simulink model "powerlib_utilityV2"  (Simulink 6.0)
settings: Solver=VariableStepDiscrete  SolverMode=SingleTasking  StartTime=0.0  StopTime=10.0  RelTol=1e-3  AbsTol=1e-6
settings Model: Creator=patrice  LastModifiedBy=batserve  ExtModeTrigMode=oneshot  ExtModeArmWhenConnect=off  ExtModeAutoUpdateStatusClock=off
settings DataIOCC: LimitDataPoints=off  SignalLoggingName=sigsOut
settings OptimizationCC: BlockReduction=off  BooleanDataType=off
settings DebuggingCC: SolverPrmCheckMsg=none  UnconnectedInputMsg=none  UnconnectedOutputMsg=none
settings HardwareCC: TargetUnknown=on
settings RTWCC: TemplateMakefile=grt_unix.tmf

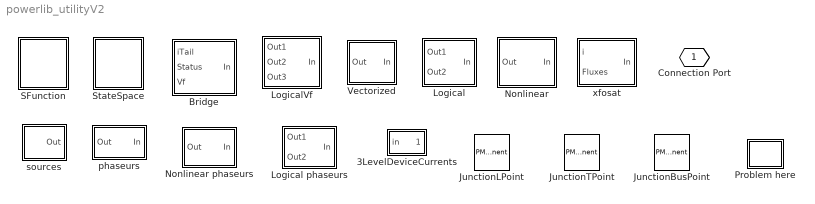
== system powerlib_utilityV2 ==
  3LevelDeviceCurrents : Subsystem  mask(Determine device currents){nb_arm=3}
      mask prompts: nb_arm "Number of arms:"
      mask init:
      | if nb_arm==1,
      |    ImesElements1=[1:3];
      |    ImesElements2=[1:10];
      | elseif nb_arm==2,
      |    ImesElements1=[1 4 2 5 3 6];
      |    ImesElements2=[1:2:19 2:2:20];
      | elseif nb_arm==3,
      |    ImesElements1=[1 4 7 2 5 8 3 6 9];
      |    ImesElements2=[1:3:28 2:3:29 3:3:30];
      | end
  Bridge : Subsystem  Orientation=left
  JunctionBusPoint : PMComponent  Tag=PoWeRsYsTeMbLoCk  PhysicalDomain=powersysdomain  LeftPortType=p1  RightPortType=p1  LConnTagsString=I1|I2  RConnTagsString=O1|O2  mask(JunctionPoint){entrees=2, sorties=2}
      mask prompts: entrees "inputs"; sorties "outputs"
      mask help: This block is used to replace the Bus Bar block from powerlib2. This block was generated by the psbupdate function. With SimPowerSystems, this block is not required. You should consider deleting this block and reconnect the lines together.
      mask init:
      | inputtags = cell(1,entrees);
      | 
      | for i=1:entrees
      | 
      | 	inputtags{i} = ['I',num2str(i)];
      | 
      | end
      | 
      | outputtags = cell(1,sorties);
      | 
      | for i=1:sorties
      | 
      | 	outputtags{i} = ['O',num2str(i)];
      | 
      | end
      | 
      | set_param(gcbh,'LConnTags',inputtags);
      | 
      | set_param(gcbh,'RConnTags',outputtags);
      mask Display:
      | color('red');
      | 
      | plot([0,100],[0,100])
      | 
      | plot([0,100],[100,0])
  JunctionLPoint : PMComponent  Tag=PoWeRsYsTeMbLoCk  PhysicalDomain=powersysdomain  LeftPortType=p1  RightPortType=p1  LConnTagsString=1  RConnTagsString=__newr0
      mask Type: JunctionPoint
      mask Description: This block is used  to replace the L connector block from powerlib2. This block was generated by the psbupdate function. With SimPowerSystems, this block is not required. You should consider deleting this block and reconnect the lines together.
      mask Display:
      | color('red');
      | 
      | plot([0,100],[0,100])
      | 
      | plot([0,100],[100,0])
  JunctionTPoint : PMComponent  Tag=PoWeRsYsTeMbLoCk  PhysicalDomain=powersysdomain  LeftPortType=p1  RightPortType=p1  LConnTagsString=1|2  RConnTagsString=__newr0
      mask Type: JunctionPoint
      mask Description: This block is used  to replace the T connector block from powerlib2. This block was generated by the psbupdate function. With SimPowerSystems, this block is not required. You should consider deleting this block and reconnect the lines together.
      mask Display:
      | color('red');
      | 
      | plot([0,100],[0,100])
      | 
      | plot([0,100],[100,0])
  Logical : Subsystem  Orientation=left
  Logical phaseurs : Subsystem  Orientation=left
  LogicalVf : Subsystem  Orientation=left
  Nonlinear : Subsystem  Orientation=left
  Nonlinear phaseurs : Subsystem  Orientation=left
  Problem here : Subsystem
      mask Display: plot([-1,1,1,-1,-1],[1,1,-1,-1,1])
  SFunction : Subsystem
  StateSpace : Subsystem
  Vectorized : Subsystem  Orientation=left
  phaseurs : Subsystem  Orientation=left
  sources : Subsystem
  xfosat : Subsystem  Orientation=left
  Connection Port : PMIOPort  Tag=PMCPort  Port=1  Side=Left

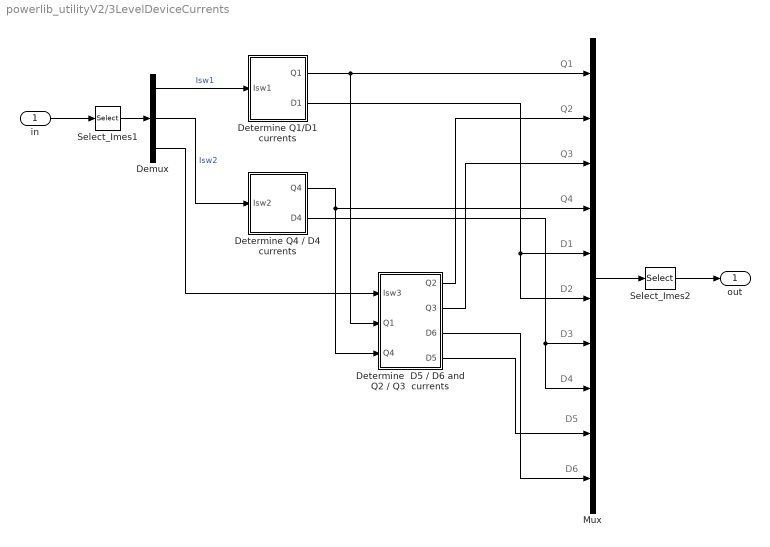
== system powerlib_utilityV2/3LevelDeviceCurrents ==
  note: Q1
  note: Q2
  note: Q3
  note: Q4
  note: D1
  note: D2
  note: D3
  note: D4
  note: D5
  note: D6
  in : Inport  Port=1  LatchInput=off
  Demux : Demux  Outputs=[nb_arm nb_arm nb_arm]
  Determine  D5 / D6 and Q2 / Q3  currents : Subsystem
  Determine Q1/D1 currents : Subsystem
  Determine Q4 / D4 currents : Subsystem
  Mux : Mux  Inputs=nb_arm*ones(10,1)
  Select_Imes1 : Selector  Elements=ImesElements1  InputPortWidth=nb_arm*3
  Select_Imes2 : Selector  Elements=ImesElements2  InputPortWidth=nb_arm*10
  out : Outport
  wires:
  Select_Imes1/1 -> Demux/1
  in/1 -> Select_Imes1/1
  Mux/1 -> Select_Imes2/1
  Select_Imes2/1 -> out/1
  Demux/1 -> Determine Q1/D1 currents/1(Isw1)  "Isw1"
  Demux/2 -> Determine Q4 / D4 currents/1(Isw2)  "Isw2"
  Demux/3 -> Determine  D5 / D6 and Q2 / Q3  currents/1(Isw3)
  Determine Q4 / D4 currents/1(Q4) -> Determine  D5 / D6 and Q2 / Q3  currents/3(Q4), Mux/4
  Determine Q1/D1 currents/1(Q1) -> Determine  D5 / D6 and Q2 / Q3  currents/2(Q1), Mux/1
  Determine  D5 / D6 and Q2 / Q3  currents/1(Q2) -> Mux/2
  Determine  D5 / D6 and Q2 / Q3  currents/2(Q3) -> Mux/3
  Determine Q1/D1 currents/2(D1) -> Mux/5, Mux/6
  Determine  D5 / D6 and Q2 / Q3  currents/3(D6) -> Mux/10
  Determine  D5 / D6 and Q2 / Q3  currents/4(D5) -> Mux/9
  Determine Q4 / D4 currents/2(D4) -> Mux/8, Mux/7

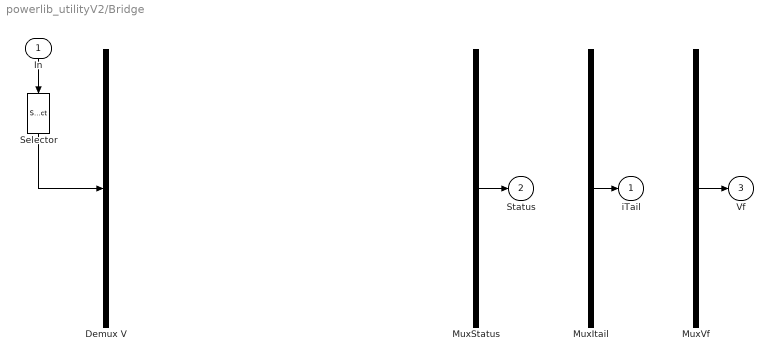
== system powerlib_utilityV2/Bridge ==
  In : Inport  Orientation=down  Port=1  LatchInput=off
  Demux V : Demux  Outputs=1
  MuxItail : Mux  Inputs=1
  MuxStatus : Mux  Inputs=1
  MuxVf : Mux  Inputs=1
  Selector : Selector  Orientation=down  InputPortWidth=1
  iTail : Outport  InitialOutput=0
  Status : Outport  Port=2  InitialOutput=0
  Vf : Outport  Port=3  InitialOutput=0
  wires:
  MuxStatus/1 -> Status/1
  MuxItail/1 -> iTail/1
  MuxVf/1 -> Vf/1
  In/1 -> Selector/1
  Selector/1 -> Demux V/1

== system powerlib_utilityV2/Logical ==
  In : Inport  Port=1  LatchInput=off
  Selector : Selector  InputPortWidth=1
  froms : Subsystem
  gotos : Subsystem
  Out1 : Outport  InitialOutput=0
  Out2 : Outport  Port=2  InitialOutput=0
  wires:
  In/1 -> Selector/1

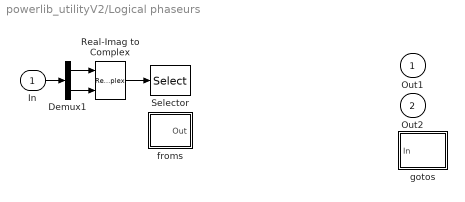
== system powerlib_utilityV2/Logical phaseurs ==
  In : Inport  Port=1  LatchInput=off
  Demux1 : Demux  Outputs=2
  Real-Imag to Complex : RealImagToComplex
  Selector : Selector  InputPortWidth=1
  froms : Subsystem
  gotos : Subsystem
  Out1 : Outport  InitialOutput=0
  Out2 : Outport  Port=2  InitialOutput=0
  wires:
  Demux1/1 -> Real-Imag to Complex/1
  Demux1/2 -> Real-Imag to Complex/2
  Real-Imag to Complex/1 -> Selector/1
  In/1 -> Demux1/1

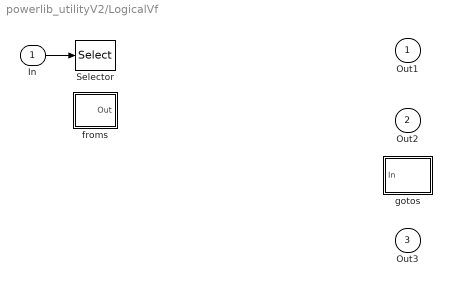
== system powerlib_utilityV2/LogicalVf ==
  In : Inport  Port=1  LatchInput=off
  Selector : Selector  InputPortWidth=1
  froms : Subsystem
  gotos : Subsystem
  Out1 : Outport  InitialOutput=0
  Out2 : Outport  Port=2  InitialOutput=0
  Out3 : Outport  Port=3  InitialOutput=0
  wires:
  In/1 -> Selector/1

== system powerlib_utilityV2/Nonlinear ==
  In : Inport  Port=1  LatchInput=off
  Demux : Demux  Outputs=1
  Mux : Mux  Inputs=1
  Selector : Selector  InputPortWidth=1
  Out : Outport  InitialOutput=0
  wires:
  In/1 -> Selector/1
  Selector/1 -> Demux/1
  Mux/1 -> Out/1

== system powerlib_utilityV2/Nonlinear phaseurs ==
  In : Inport  Port=1  LatchInput=off
  Demux : Demux  Outputs=1
  Demux1 : Demux  Outputs=2
  Mux : Mux  Inputs=1
  Real-Imag to Complex : RealImagToComplex
  Selector : Selector  InputPortWidth=1
  Out : Outport  InitialOutput=0
  wires:
  Mux/1 -> Out/1
  Selector/1 -> Demux/1
  Demux1/1 -> Real-Imag to Complex/1
  Demux1/2 -> Real-Imag to Complex/2
  In/1 -> Demux1/1
  Real-Imag to Complex/1 -> Selector/1

== system powerlib_utilityV2/Problem here ==
  note: This block identifies a connection problem
      | during the update of the model

== system powerlib_utilityV2/SFunction ==
  phaseurs : Subsystem
      mask init:
      | H=0;Rswitch=1;
  phaseursNoVf : Subsystem
      mask init:
      | H=0;Rswitch=1;
  structure : Subsystem
      mask init:
      | A=0;B=0;C=0;D=0;x0=0;Rswitch=1;TypeSwitch=0;Ts=0;YSwitchCurrent=-1;
  structureNoVf : Subsystem
      mask init:
      | A=0;B=0;C=0;D=0;x0=0;Rswitch=1;TypeSwitch=0;Ts=0;YSwitchCurrent=-1;

== system powerlib_utilityV2/StateSpace ==
  phaseurs : Subsystem
      mask init:
      | H=0;Rswitch=1;
  phaseursNoVf : Subsystem
      mask init:
      | H=0;Rswitch=1;
  structure1 : Subsystem
      mask init:
      | A=0;B=0;C=0;D=0;x0=0;Rswitch=1;TypeSwitch=0;Ts=0;
  structure1Discrete : Subsystem
      mask init:
      | A=0;B=0;C=0;D=0;x0=0;Rswitch=1;TypeSwitch=0;Ts=0;
  structure2 : Subsystem
      mask init:
      | A=0;B=0;C=0;D=0;x0=0;Rswitch=1;TypeSwitch=0;Ts=0;
  structure2Discrete : Subsystem
      mask init:
      | A=0;B=0;C=0;D=0;x0=0;Rswitch=1;TypeSwitch=0;Ts=0;

== system powerlib_utilityV2/Vectorized ==
  In : Inport  Port=1  LatchInput=off
  Selector : Selector  InputPortWidth=1
  froms : Subsystem
  gotos : Subsystem
  Out : Outport  InitialOutput=0
  wires:
  In/1 -> Selector/1

== system powerlib_utilityV2/phaseurs ==
  In : Inport  Port=1  LatchInput=off
  Demux : Demux  Outputs=1
  Demux1 : Demux  Outputs=2
  Mux : Mux  Inputs=1
  Real-Imag to Complex : RealImagToComplex
  Selector : Selector  InputPortWidth=1
  Out : Outport  InitialOutput=0
  wires:
  Mux/1 -> Out/1
  Selector/1 -> Demux/1
  Demux1/1 -> Real-Imag to Complex/1
  Demux1/2 -> Real-Imag to Complex/2
  Real-Imag to Complex/1 -> Selector/1
  In/1 -> Demux1/1

== system powerlib_utilityV2/sources ==
  Mux : Mux  Inputs=1
  Selector : Selector  InputPortWidth=1
  Out : Outport  InitialOutput=0
  wires:
  Mux/1 -> Selector/1
  Selector/1 -> Out/1

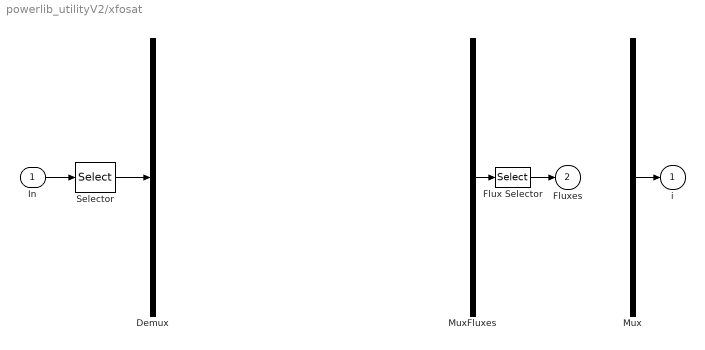
== system powerlib_utilityV2/xfosat ==
  In : Inport  Port=1  LatchInput=off
  Demux : Demux  Outputs=1
  Flux Selector : Selector  InputPortWidth=1
  Mux : Mux  Inputs=1
  MuxFluxes : Mux  Inputs=1
  Selector : Selector  InputPortWidth=1
  i : Outport  InitialOutput=0
  Fluxes : Outport  Port=2  InitialOutput=0
  wires:
  In/1 -> Selector/1
  Selector/1 -> Demux/1
  Mux/1 -> i/1
  MuxFluxes/1 -> Flux Selector/1
  Flux Selector/1 -> Fluxes/1

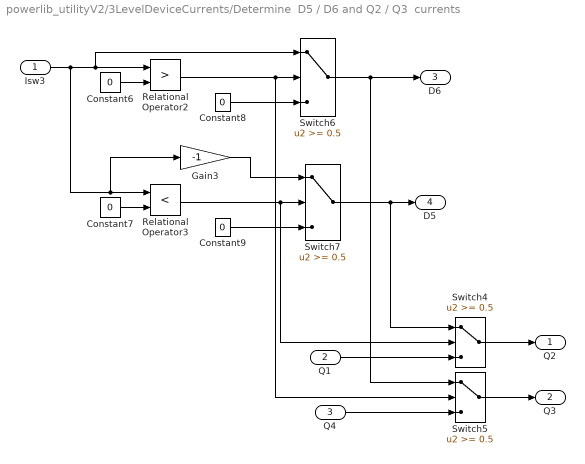
== system powerlib_utilityV2/3LevelDeviceCurrents/Determine  D5 / D6 and Q2 / Q3  currents ==
  Isw3 : Inport  Port=1  LatchInput=off
  Q1 : Inport  Port=2  LatchInput=off
  Q4 : Inport  Port=3  LatchInput=off
  Constant{6..9} (4 alike) : Constant  Value=0
  Gain3 : Gain  Gain=-1  SaturateOnIntegerOverflow=on
  Relational Operator2 : RelationalOperator  Operator=>  InputSameDT=on
  Relational Operator3 : RelationalOperator  Operator=<  InputSameDT=on
  Switch{4..7} (4 alike) : Switch  Threshold=0.5  SaturateOnIntegerOverflow=on  InputSameDT=on
  Q2 : Outport
  Q3 : Outport  Port=2
  D6 : Outport  Port=3
  D5 : Outport  Port=4
  wires:
  Gain3/1 -> Switch7/1
  Constant9/1 -> Switch7/3
  Constant8/1 -> Switch6/3
  Relational Operator3/1 -> Switch7/2, Switch4/2
  Isw3/1 -> Relational Operator2/1, Switch6/1, Relational Operator3/1, Gain3/1
  Relational Operator2/1 -> Switch6/2, Switch5/2
  Constant7/1 -> Relational Operator3/2
  Constant6/1 -> Relational Operator2/2
  Switch4/1 -> Q2/1
  Switch5/1 -> Q3/1
  Switch6/1 -> D6/1, Switch5/1
  Switch7/1 -> D5/1, Switch4/1
  Q1/1 -> Switch4/3
  Q4/1 -> Switch5/3

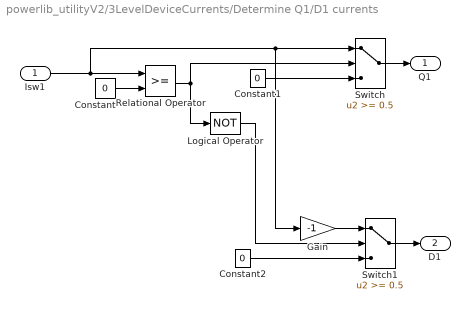
== system powerlib_utilityV2/3LevelDeviceCurrents/Determine Q1/D1 currents ==
  Isw1 : Inport  Port=1  LatchInput=off
  Constant : Constant  Value=0
  Constant1 : Constant  Value=0
  Constant2 : Constant  Value=0
  Gain : Gain  Gain=-1  SaturateOnIntegerOverflow=on
  Logical Operator : Logic  Operator=NOT
  Relational Operator : RelationalOperator  InputSameDT=on
  Switch : Switch  Threshold=0.5  SaturateOnIntegerOverflow=on  InputSameDT=on
  Switch1 : Switch  Threshold=0.5  SaturateOnIntegerOverflow=on  InputSameDT=on
  Q1 : Outport
  D1 : Outport  Port=2
  wires:
  Gain/1 -> Switch1/1
  Logical Operator/1 -> Switch1/2
  Constant2/1 -> Switch1/3
  Relational Operator/1 -> Logical Operator/1, Switch/2
  Constant1/1 -> Switch/3
  Constant/1 -> Relational Operator/2
  Isw1/1 -> Relational Operator/1, Switch/1, Gain/1
  Switch/1 -> Q1/1
  Switch1/1 -> D1/1

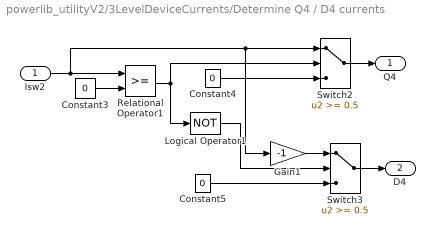
== system powerlib_utilityV2/3LevelDeviceCurrents/Determine Q4 / D4 currents ==
  Isw2 : Inport  Port=1  LatchInput=off
  Constant3 : Constant  Value=0
  Constant4 : Constant  Value=0
  Constant5 : Constant  Value=0
  Gain1 : Gain  Gain=-1  SaturateOnIntegerOverflow=on
  Logical Operator1 : Logic  Operator=NOT
  Relational Operator1 : RelationalOperator  InputSameDT=on
  Switch2 : Switch  Threshold=0.5  SaturateOnIntegerOverflow=on  InputSameDT=on
  Switch3 : Switch  Threshold=0.5  SaturateOnIntegerOverflow=on  InputSameDT=on
  Q4 : Outport
  D4 : Outport  Port=2
  wires:
  Gain1/1 -> Switch3/1
  Logical Operator1/1 -> Switch3/2
  Constant5/1 -> Switch3/3
  Relational Operator1/1 -> Switch2/2, Logical Operator1/1
  Constant4/1 -> Switch2/3
  Constant3/1 -> Relational Operator1/2
  Isw2/1 -> Gain1/1, Switch2/1, Relational Operator1/1
  Switch2/1 -> Q4/1
  Switch3/1 -> D4/1

== system powerlib_utilityV2/Logical/froms ==
  Mux : Mux  Inputs=1
  Out : Outport  InitialOutput=0
  wires:
  Mux/1 -> Out/1

== system powerlib_utilityV2/Logical/gotos ==
  In : Inport  Port=1  LatchInput=off
  Demux : Demux  Outputs=1
  Selector : Selector  InputPortWidth=1
  wires:
  Selector/1 -> Demux/1
  In/1 -> Selector/1

== system powerlib_utilityV2/Logical phaseurs/froms ==
  Mux : Mux  Inputs=1
  Out : Outport  InitialOutput=0
  wires:
  Mux/1 -> Out/1

== system powerlib_utilityV2/Logical phaseurs/gotos ==
  In : Inport  Port=1  LatchInput=off
  Demux : Demux  Outputs=1
  Selector : Selector  InputPortWidth=1
  wires:
  In/1 -> Selector/1
  Selector/1 -> Demux/1

== system powerlib_utilityV2/LogicalVf/froms ==
  Mux : Mux  Inputs=1
  Out : Outport  InitialOutput=0
  wires:
  Mux/1 -> Out/1

== system powerlib_utilityV2/LogicalVf/gotos ==
  In : Inport  Port=1  LatchInput=off
  Demux : Demux  Outputs=1
  Selector : Selector  InputPortWidth=1
  wires:
  In/1 -> Selector/1
  Selector/1 -> Demux/1

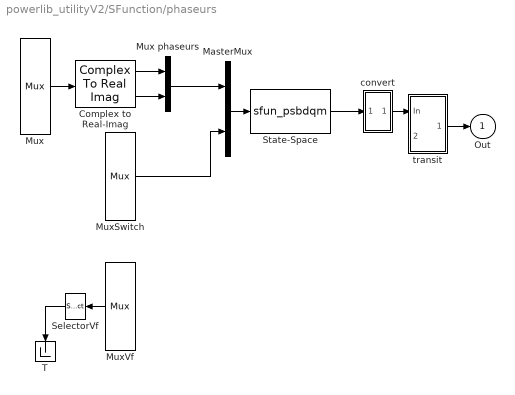
== system powerlib_utilityV2/SFunction/phaseurs ==
  Complex to Real-Imag : ComplexToRealImag
  MasterMux : Mux  Inputs=2
  Mux : Mux  Inputs=1
  Mux phaseurs : Mux  Inputs=2
  MuxSwitch : Mux  Inputs=1
  MuxVf : Mux  Orientation=left  Inputs=1
  SelectorVf : Selector  Orientation=left  InputPortWidth=1
  State-Space : S-Function  FunctionName=sfun_psbdqm  Parameters=H, Rswitch
  T : Terminator
      settings: Orientation=down
  convert : Subsystem
  transit : Subsystem
  Out : Outport  InitialOutput=0
  wires:
  SelectorVf/1 -> T/1
  MuxVf/1 -> SelectorVf/1
  MasterMux/1 -> State-Space/1
  transit/1(Out) -> Out/1
  Mux/1 -> Complex to Real-Imag/1
  State-Space/1 -> convert/1(In1)
  Complex to Real-Imag/2 -> Mux phaseurs/2
  Complex to Real-Imag/1 -> Mux phaseurs/1
  Mux phaseurs/1 -> MasterMux/1
  MuxSwitch/1 -> MasterMux/2
  convert/1(Out1) -> transit/1(In)

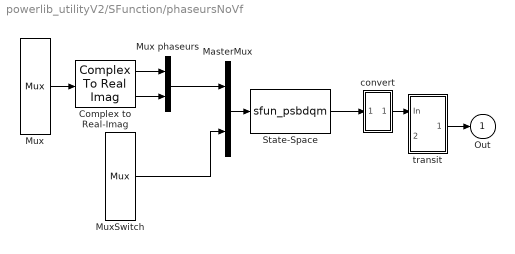
== system powerlib_utilityV2/SFunction/phaseursNoVf ==
  Complex to Real-Imag : ComplexToRealImag
  MasterMux : Mux  Inputs=2
  Mux : Mux  Inputs=1
  Mux phaseurs : Mux  Inputs=2
  MuxSwitch : Mux  Inputs=1
  State-Space : S-Function  FunctionName=sfun_psbdqm  Parameters=H, Rswitch
  convert : Subsystem
  transit : Subsystem
  Out : Outport  InitialOutput=0
  wires:
  convert/1(Out1) -> transit/1(In)
  MuxSwitch/1 -> MasterMux/2
  Mux phaseurs/1 -> MasterMux/1
  Complex to Real-Imag/1 -> Mux phaseurs/1
  Complex to Real-Imag/2 -> Mux phaseurs/2
  State-Space/1 -> convert/1(In1)
  Mux/1 -> Complex to Real-Imag/1
  transit/1(Out) -> Out/1
  MasterMux/1 -> State-Space/1

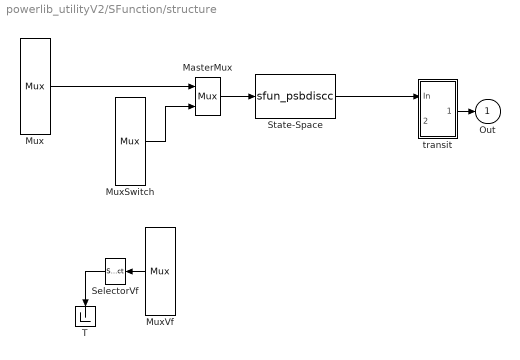
== system powerlib_utilityV2/SFunction/structure ==
  MasterMux : Mux  Inputs=2
  Mux : Mux  Inputs=1
  MuxSwitch : Mux  Inputs=1
  MuxVf : Mux  Orientation=left  Inputs=1
  SelectorVf : Selector  Orientation=left  InputPortWidth=1
  State-Space : S-Function  FunctionName=sfun_psbdiscc  Parameters=A,B,C,D,x0,Rswitch,TypeSwitch,Ts,YSwitchCurrent
  T : Terminator
      settings: Orientation=down
  transit : Subsystem
  Out : Outport  InitialOutput=0
  wires:
  transit/1(Out) -> Out/1
  State-Space/1 -> transit/1(In)
  MasterMux/1 -> State-Space/1
  MuxSwitch/1 -> MasterMux/2
  Mux/1 -> MasterMux/1
  MuxVf/1 -> SelectorVf/1
  SelectorVf/1 -> T/1

== system powerlib_utilityV2/SFunction/structureNoVf ==
  MasterMux : Mux  Inputs=2
  Mux : Mux  Inputs=1
  MuxSwitch : Mux  Inputs=1
  State-Space : S-Function  FunctionName=sfun_psbdiscc  Parameters=A,B,C,D,x0,Rswitch,TypeSwitch,Ts,YSwitchCurrent
  transit : Subsystem
  Out : Outport  InitialOutput=0
  wires:
  Mux/1 -> MasterMux/1
  MuxSwitch/1 -> MasterMux/2
  MasterMux/1 -> State-Space/1
  State-Space/1 -> transit/1(In)
  transit/1(Out) -> Out/1

== system powerlib_utilityV2/StateSpace/phaseurs ==
  Complex to Real-Imag : ComplexToRealImag
  Mux : Mux  Inputs=1
  Mux phaseurs : Mux  Inputs=2
  State-Space : S-Function  FunctionName=sfun_psbdqm  Parameters=H, Rswitch
  convert : Subsystem
  transit : Subsystem
  Out : Outport  InitialOutput=0
  wires:
  Mux phaseurs/1 -> State-Space/1
  Complex to Real-Imag/1 -> Mux phaseurs/1
  Complex to Real-Imag/2 -> Mux phaseurs/2
  State-Space/1 -> convert/1(In1)
  Mux/1 -> Complex to Real-Imag/1
  transit/1(Out) -> Out/1
  convert/1(Out1) -> transit/1(In)

== system powerlib_utilityV2/StateSpace/phaseursNoVf ==
  Complex to Real-Imag : ComplexToRealImag
  Mux : Mux  Inputs=1
  Mux phaseurs : Mux  Inputs=2
  State-Space : S-Function  FunctionName=sfun_psbdqm  Parameters=H, Rswitch
  convert : Subsystem
  transit : Subsystem
  Out : Outport  InitialOutput=0
  wires:
  convert/1(Out1) -> transit/1(In)
  transit/1(Out) -> Out/1
  Mux/1 -> Complex to Real-Imag/1
  State-Space/1 -> convert/1(In1)
  Complex to Real-Imag/2 -> Mux phaseurs/2
  Complex to Real-Imag/1 -> Mux phaseurs/1
  Mux phaseurs/1 -> State-Space/1

== system powerlib_utilityV2/StateSpace/structure1 ==
  Ground : Ground
  State-Space : StateSpace  A=A  B=B  C=C  D=D  X0=x0
  transit : Subsystem
  Out : Outport  InitialOutput=0
  wires:
  Ground/1 -> State-Space/1
  transit/1(Out) -> Out/1
  State-Space/1 -> transit/1(In)

== system powerlib_utilityV2/StateSpace/structure1Discrete ==
  Ground : Ground
  State-Space : DiscreteStateSpace  A=A  B=B  C=C  D=D  X0=x0  SampleTime=Ts
  transit : Subsystem
  Out : Outport  InitialOutput=0
  wires:
  State-Space/1 -> transit/1(In)
  transit/1(Out) -> Out/1
  Ground/1 -> State-Space/1

== system powerlib_utilityV2/StateSpace/structure2 ==
  Mux : Mux  Inputs=1
  State-Space : StateSpace  A=A  B=B  C=C  D=D  X0=x0
  transit : Subsystem
  Out : Outport  InitialOutput=0
  wires:
  Mux/1 -> State-Space/1
  transit/1(Out) -> Out/1
  State-Space/1 -> transit/1(In)

== system powerlib_utilityV2/StateSpace/structure2Discrete ==
  Mux : Mux  Inputs=1
  State-Space : DiscreteStateSpace  A=A  B=B  C=C  D=D  X0=x0  SampleTime=Ts
  transit : Subsystem
  Out : Outport  InitialOutput=0
  wires:
  State-Space/1 -> transit/1(In)
  transit/1(Out) -> Out/1
  Mux/1 -> State-Space/1

== system powerlib_utilityV2/Vectorized/froms ==
  Mux : Mux  Inputs=1
  Out : Outport  InitialOutput=0
  wires:
  Mux/1 -> Out/1

== system powerlib_utilityV2/Vectorized/gotos ==
  In : Inport  Port=1  LatchInput=off
  Demux : Demux  Outputs=1
  Selector : Selector  InputPortWidth=1
  wires:
  In/1 -> Selector/1
  Selector/1 -> Demux/1

== system powerlib_utilityV2/SFunction/phaseurs/convert ==
  In1 : Inport  Port=1  LatchInput=off
  Demux1 : Demux  Outputs=2
  Real-Imag to Complex : RealImagToComplex
  Out1 : Outport
  wires:
  Demux1/1 -> Real-Imag to Complex/1
  Demux1/2 -> Real-Imag to Complex/2
  Real-Imag to Complex/1 -> Out1/1
  In1/1 -> Demux1/1

== system powerlib_utilityV2/SFunction/phaseurs/transit ==
  In : Inport  Port=1  LatchInput=off
  signals : Inport  Port=2  LatchInput=off
  Demux : Demux  Outputs=1
  Selector : Selector  InputPortWidth=1
  Terminator : Terminator
      settings: Orientation=down
  Out : Outport  Orientation=left  InitialOutput=0
  wires:
  signals/1 -> Terminator/1
  In/1 -> Selector/1
  Selector/1 -> Demux/1

== system powerlib_utilityV2/SFunction/phaseursNoVf/convert ==
  In1 : Inport  Port=1  LatchInput=off
  Demux1 : Demux  Outputs=2
  Real-Imag to Complex : RealImagToComplex
  Out1 : Outport
  wires:
  In1/1 -> Demux1/1
  Real-Imag to Complex/1 -> Out1/1
  Demux1/2 -> Real-Imag to Complex/2
  Demux1/1 -> Real-Imag to Complex/1

== system powerlib_utilityV2/SFunction/phaseursNoVf/transit ==
  In : Inport  Port=1  LatchInput=off
  signals : Inport  Port=2  LatchInput=off
  Demux : Demux  Outputs=1
  Selector : Selector  InputPortWidth=1
  Terminator : Terminator
      settings: Orientation=down
  Out : Outport  Orientation=left  InitialOutput=0
  wires:
  Selector/1 -> Demux/1
  In/1 -> Selector/1
  signals/1 -> Terminator/1

== system powerlib_utilityV2/SFunction/structure/transit ==
  In : Inport  Port=1  LatchInput=off
  signals : Inport  Port=2  LatchInput=off
  Demux : Demux  Outputs=1
  Selector : Selector  InputPortWidth=1
  Terminator : Terminator
      settings: Orientation=down
  Out : Outport  Orientation=left  InitialOutput=0
  wires:
  In/1 -> Selector/1
  Selector/1 -> Demux/1
  signals/1 -> Terminator/1

== system powerlib_utilityV2/SFunction/structureNoVf/transit ==
  In : Inport  Port=1  LatchInput=off
  signals : Inport  Port=2  LatchInput=off
  Demux : Demux  Outputs=1
  Selector : Selector  InputPortWidth=1
  Terminator : Terminator
      settings: Orientation=down
  Out : Outport  Orientation=left  InitialOutput=0
  wires:
  signals/1 -> Terminator/1
  Selector/1 -> Demux/1
  In/1 -> Selector/1

== system powerlib_utilityV2/StateSpace/phaseurs/convert ==
  In1 : Inport  Port=1  LatchInput=off
  Demux1 : Demux  Outputs=2
  Real-Imag to Complex : RealImagToComplex
  Out1 : Outport
  wires:
  Demux1/2 -> Real-Imag to Complex/2
  Demux1/1 -> Real-Imag to Complex/1
  Real-Imag to Complex/1 -> Out1/1
  In1/1 -> Demux1/1

== system powerlib_utilityV2/StateSpace/phaseurs/transit ==
  In : Inport  Port=1  LatchInput=off
  signals : Inport  Port=2  LatchInput=off
  Demux : Demux  Outputs=1
  Selector : Selector  InputPortWidth=2
  Terminator : Terminator
      settings: Orientation=down
  Out : Outport  Orientation=left  InitialOutput=0
  wires:
  Selector/1 -> Demux/1
  In/1 -> Selector/1
  signals/1 -> Terminator/1

== system powerlib_utilityV2/StateSpace/phaseursNoVf/convert ==
  In1 : Inport  Port=1  LatchInput=off
  Demux1 : Demux  Outputs=2
  Real-Imag to Complex : RealImagToComplex
  Out1 : Outport
  wires:
  In1/1 -> Demux1/1
  Real-Imag to Complex/1 -> Out1/1
  Demux1/1 -> Real-Imag to Complex/1
  Demux1/2 -> Real-Imag to Complex/2

== system powerlib_utilityV2/StateSpace/phaseursNoVf/transit ==
  In : Inport  Port=1  LatchInput=off
  signals : Inport  Port=2  LatchInput=off
  Demux : Demux  Outputs=1
  Selector : Selector  InputPortWidth=2
  Terminator : Terminator
      settings: Orientation=down
  Out : Outport  Orientation=left  InitialOutput=0
  wires:
  signals/1 -> Terminator/1
  In/1 -> Selector/1
  Selector/1 -> Demux/1

== system powerlib_utilityV2/StateSpace/structure1/transit ==
  In : Inport  Port=1  LatchInput=off
  signals : Inport  Port=2  LatchInput=off
  Demux : Demux  Outputs=1
  Selector : Selector  InputPortWidth=1
  Terminator : Terminator
      settings: Orientation=down
  Out : Outport  Orientation=left  InitialOutput=0
  wires:
  signals/1 -> Terminator/1
  Selector/1 -> Demux/1
  In/1 -> Selector/1

== system powerlib_utilityV2/StateSpace/structure1Discrete/transit ==
  In : Inport  Port=1  LatchInput=off
  signals : Inport  Port=2  LatchInput=off
  Demux : Demux  Outputs=1
  Selector : Selector  InputPortWidth=1
  Terminator : Terminator
      settings: Orientation=down
  Out : Outport  Orientation=left  InitialOutput=0
  wires:
  signals/1 -> Terminator/1
  Selector/1 -> Demux/1
  In/1 -> Selector/1

== system powerlib_utilityV2/StateSpace/structure2/transit ==
  In : Inport  Port=1  LatchInput=off
  signals : Inport  Port=2  LatchInput=off
  Demux : Demux  Outputs=1
  Selector : Selector  InputPortWidth=1
  Terminator : Terminator
      settings: Orientation=down
  Out : Outport  Orientation=left  InitialOutput=0
  wires:
  signals/1 -> Terminator/1
  Selector/1 -> Demux/1
  In/1 -> Selector/1

== system powerlib_utilityV2/StateSpace/structure2Discrete/transit ==
  In : Inport  Port=1  LatchInput=off
  signals : Inport  Port=2  LatchInput=off
  Demux : Demux  Outputs=1
  Selector : Selector  InputPortWidth=1
  Terminator : Terminator
      settings: Orientation=down
  Out : Outport  Orientation=left  InitialOutput=0
  wires:
  signals/1 -> Terminator/1
  Selector/1 -> Demux/1
  In/1 -> Selector/1
